simulink model "PhoenixKalman"  (R2016a)
settings: Solver=VariableStepAuto  StartTime=Seconds(firstPoint,1)  StopTime=Seconds(lastPoint,1)  RelTol=1e-3
libraries: aerolibactuator x4, aerolibanim x2, aerolib6dof2 x1, aerolibconvert2 x1
settings Model: Creator=GusBus  LastModifiedBy=GusBus
settings GRTTargetCC: GeneratePreprocessorConditionals=Use local settings

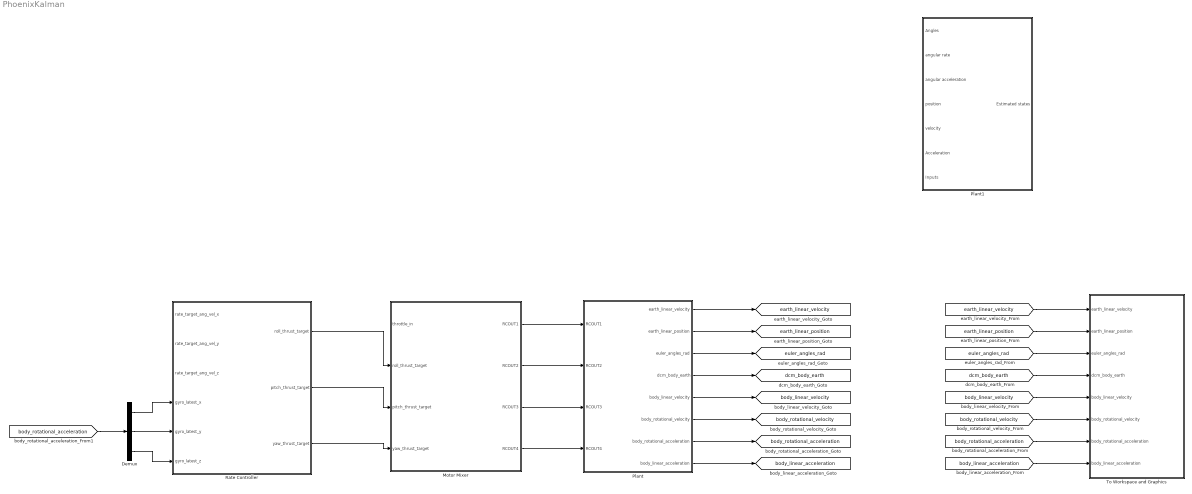
== system PhoenixKalman ==
  Demux : Demux  Outputs=3
  Motor Mixer : MATLAB Function  TreatAsAtomicUnit=on
  Plant : Subsystem
  Plant1 : Subsystem
  Rate Controller : MATLAB Function  TreatAsAtomicUnit=on
  To Workspace and Graphics : Subsystem
  tag scope: body_linear_acceleration=global, body_linear_velocity=global, body_rotational_acceleration=global, body_rotational_velocity=global, dcm_body_earth=global, earth_linear_position=global, earth_linear_velocity=global, euler_angles_rad=global
  wires:
  [body_rotational_velocity] -> To Workspace and Graphics/6(body_rotational_velocity)
  [body_linear_acceleration] -> To Workspace and Graphics/8(body_linear_acceleration)
  [body_rotational_acceleration] -> To Workspace and Graphics/7(body_rotational_acceleration)
  [body_linear_velocity] -> To Workspace and Graphics/5(body_linear_velocity)
  [dcm_body_earth] -> To Workspace and Graphics/4(dcm_body_earth)
  [euler_angles_rad] -> To Workspace and Graphics/3(euler_angles_rad)
  [earth_linear_position] -> To Workspace and Graphics/2(earth_linear_position)
  [earth_linear_velocity] -> To Workspace and Graphics/1(earth_linear_velocity)
  Plant/1(earth_linear_velocity) -> [earth_linear_velocity]
  Plant/2(earth_linear_position) -> [earth_linear_position]
  Plant/3(euler_angles_rad) -> [euler_angles_rad]
  Plant/4(dcm_body_earth) -> [dcm_body_earth]
  Plant/5(body_linear_velocity) -> [body_linear_velocity]
  Plant/6(body_rotational_velocity) -> [body_rotational_velocity]
  Plant/7(body_rotational_acceleration) -> [body_rotational_acceleration]
  Plant/8(body_linear_acceleration) -> [body_linear_acceleration]
  Motor Mixer/1(RCOUT1) -> Plant/1(RCOUT1)
  Motor Mixer/2(RCOUT2) -> Plant/2(RCOUT2)
  Motor Mixer/3(RCOUT3) -> Plant/3(RCOUT3)
  Motor Mixer/4(RCOUT4) -> Plant/4(RCOUT4)
  Rate Controller/1(roll_thrust_target) -> Motor Mixer/2(roll_thrust_target)
  Rate Controller/2(pitch_thrust_target) -> Motor Mixer/3(pitch_thrust_target)
  Rate Controller/3(yaw_thrust_target) -> Motor Mixer/4(yaw_thrust_target)
  Demux/1 -> Rate Controller/4(gyro_latest_x)
  Demux/2 -> Rate Controller/5(gyro_latest_y)
  Demux/3 -> Rate Controller/6(gyro_latest_z)
  [body_rotational_acceleration] -> Demux/1

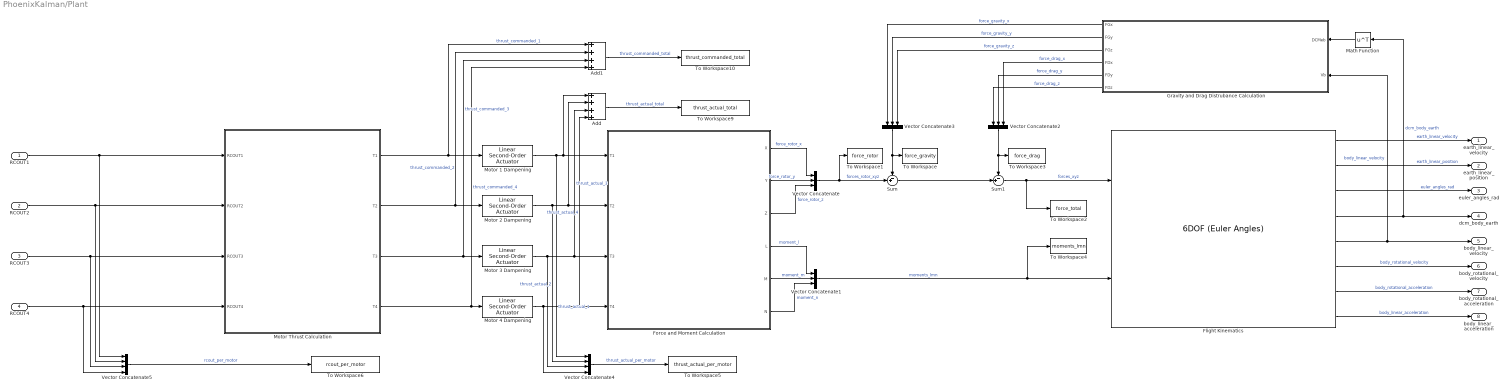
== system PhoenixKalman/Plant ==
  RCOUT1 : Inport
  RCOUT2 : Inport  Port=2
  RCOUT3 : Inport  Port=3
  RCOUT4 : Inport  Port=4
  Add : Sum  Inputs=++++
  Add1 : Sum  Inputs=++++
  Flight Kinematics : aerolib6dof2/6DOF (Euler Angles)  units=Metric (MKS)  mtype=Fixed  rep=Euler Angles  xme_0=[0 0 0]  Vm_0=[0 0 0]  eul_0=InitialAngles  pm_0=InitialRate  mass_0=2.2  mass_e=0.5  mass_f=2.0  inertia=[0.5 0 0; 0 0.5 0; 0 0 0.85]  inertia_e=eye(3)  inertia_f=2*eye(3)  k_quat=1.0  vre_flag=on
  Force and Moment Calculation : MATLAB Function  TreatAsAtomicUnit=on
  Gravity and Drag Distrubance Calculation : MATLAB Function  TreatAsAtomicUnit=on
  Math Function : Math  Operator=transpose  SaturateOnIntegerOverflow=on
  Motor 1 Dampening : aerolibactuator/Linear Second-Order Actuator  wn_fin=500  z_fin=1  fin_act_0=0  fin_act_vel=0
  Motor 2 Dampening : aerolibactuator/Linear Second-Order Actuator  wn_fin=500  z_fin=1  fin_act_0=0  fin_act_vel=0
  Motor 3 Dampening : aerolibactuator/Linear Second-Order Actuator  wn_fin=500  z_fin=1  fin_act_0=0  fin_act_vel=0
  Motor 4 Dampening : aerolibactuator/Linear Second-Order Actuator  wn_fin=500  z_fin=1  fin_act_0=0  fin_act_vel=0
  Motor Thrust Calculation : MATLAB Function  TreatAsAtomicUnit=on
  Sum : Sum  Inputs=-+|
  Sum1 : Sum  Inputs=-+|
  To Workspace : ToWorkspace  VariableName=force_gravity  SampleTime=-1
  To Workspace1 : ToWorkspace  VariableName=force_rotor  SampleTime=-1
  To Workspace10 : ToWorkspace  VariableName=thrust_commanded_total  SampleTime=-1
  To Workspace2 : ToWorkspace  VariableName=force_total  SampleTime=-1
  To Workspace3 : ToWorkspace  VariableName=force_drag  SampleTime=-1
  To Workspace4 : ToWorkspace  VariableName=moments_lmn  SampleTime=-1
  To Workspace5 : ToWorkspace  VariableName=thrust_actual_per_motor  SampleTime=-1
  To Workspace6 : ToWorkspace  VariableName=rcout_per_motor  SampleTime=-1
  To Workspace9 : ToWorkspace  VariableName=thrust_actual_total  SampleTime=-1
  Vector Concatenate{,1..3} (4 alike) : Concatenate  NumInputs=3
  Vector Concatenate4 : Concatenate  NumInputs=4
  Vector Concatenate5 : Concatenate  NumInputs=4
  earth_linear_velocity : Outport
  earth_linear_position : Outport  Port=2
  euler_angles_rad : Outport  Port=3
  dcm_body_earth : Outport  Port=4
  body_linear_velocity : Outport  Port=5
  body_rotational_velocity : Outport  Port=6
  body_rotational_acceleration : Outport  Port=7
  body_linear_acceleration : Outport  Port=8
  wires:
  Force and Moment Calculation/2(Y) -> Vector Concatenate/2  "force_rotor_y"
  Force and Moment Calculation/1(X) -> Vector Concatenate/1  "force_rotor_x"
  Force and Moment Calculation/3(Z) -> Vector Concatenate/3  "force_rotor_z"
  Force and Moment Calculation/6(N) -> Vector Concatenate1/3  "moment_n"
  Force and Moment Calculation/4(L) -> Vector Concatenate1/1  "moment_l"
  Motor Thrust Calculation/2(T2) -> Add1/2, Motor 2 Dampening/1  "thrust_commanded_2"
  Vector Concatenate1/1 -> To Workspace4/1, Flight Kinematics/2  "moments_lmn"
  Force and Moment Calculation/5(M) -> Vector Concatenate1/2  "moment_m"
  Motor 2 Dampening/1 -> Vector Concatenate4/2, Add/2, Force and Moment Calculation/2(T2)  "thrust_actual_2"
  Vector Concatenate/1 -> Sum/2, To Workspace1/1  "forces_rotor_xyz"
  Gravity and Drag Distrubance Calculation/6(FDz) -> Vector Concatenate2/1  "force_drag_z"
  Vector Concatenate3/1 -> To Workspace/1, Sum/1
  Add/1 -> To Workspace9/1  "thrust_actual_total"
  Gravity and Drag Distrubance Calculation/2(FGy) -> Vector Concatenate3/2  "force_gravity_y"
  Flight Kinematics/7 -> body_rotational_acceleration/1  "body_rotational_acceleration"
  Sum/1 -> Sum1/2
  Flight Kinematics/3 -> euler_angles_rad/1  "euler_angles_rad"
  Flight Kinematics/4 -> Math Function/1, dcm_body_earth/1  "dcm_body_earth"
  Vector Concatenate2/1 -> To Workspace3/1, Sum1/1
  Gravity and Drag Distrubance Calculation/1(FGx) -> Vector Concatenate3/1  "force_gravity_x"
  Motor Thrust Calculation/1(T1) -> Add1/1, Motor 1 Dampening/1  "thrust_commanded_1"
  Math Function/1 -> Gravity and Drag Distrubance Calculation/1(DCMeb)
  Add1/1 -> To Workspace10/1  "thrust_commanded_total"
  Motor Thrust Calculation/3(T3) -> Add1/3, Motor 3 Dampening/1  "thrust_commanded_3"
  Flight Kinematics/6 -> body_rotational_velocity/1  "body_rotational_velocity"
  Flight Kinematics/5 -> Gravity and Drag Distrubance Calculation/2(Vb), body_linear_velocity/1  "body_linear_velocity"
  Motor 1 Dampening/1 -> Vector Concatenate4/1, Add/1, Force and Moment Calculation/1(T1)  "thrust_actual_1"
  Motor 4 Dampening/1 -> Vector Concatenate4/4, Add/4, Force and Moment Calculation/4(T4)  "thrust_actual_4"
  Sum1/1 -> Flight Kinematics/1, To Workspace2/1  "forces_xyz"
  Gravity and Drag Distrubance Calculation/3(FGz) -> Vector Concatenate3/3  "force_gravity_z"
  Flight Kinematics/1 -> earth_linear_velocity/1  "earth_linear_velocity"
  Motor Thrust Calculation/4(T4) -> Add1/4, Motor 4 Dampening/1  "thrust_commanded_4"
  Gravity and Drag Distrubance Calculation/4(FDx) -> Vector Concatenate2/3  "force_drag_x"
  Gravity and Drag Distrubance Calculation/5(FDy) -> Vector Concatenate2/2  "force_drag_y"
  Flight Kinematics/8 -> body_linear_acceleration/1  "body_linear_acceleration"
  Motor 3 Dampening/1 -> Vector Concatenate4/3, Add/3, Force and Moment Calculation/3(T3)  "thrust_actual_3"
  Vector Concatenate4/1 -> To Workspace5/1  "thrust_actual_per_motor"
  Vector Concatenate5/1 -> To Workspace6/1  "rcout_per_motor"
  RCOUT1/1 -> Vector Concatenate5/1, Motor Thrust Calculation/1(RCOUT1)
  Flight Kinematics/2 -> earth_linear_position/1  "earth_linear_position"
  RCOUT2/1 -> Vector Concatenate5/2, Motor Thrust Calculation/2(RCOUT2)
  RCOUT4/1 -> Vector Concatenate5/4, Motor Thrust Calculation/4(RCOUT4)
  RCOUT3/1 -> Vector Concatenate5/3, Motor Thrust Calculation/3(RCOUT3)

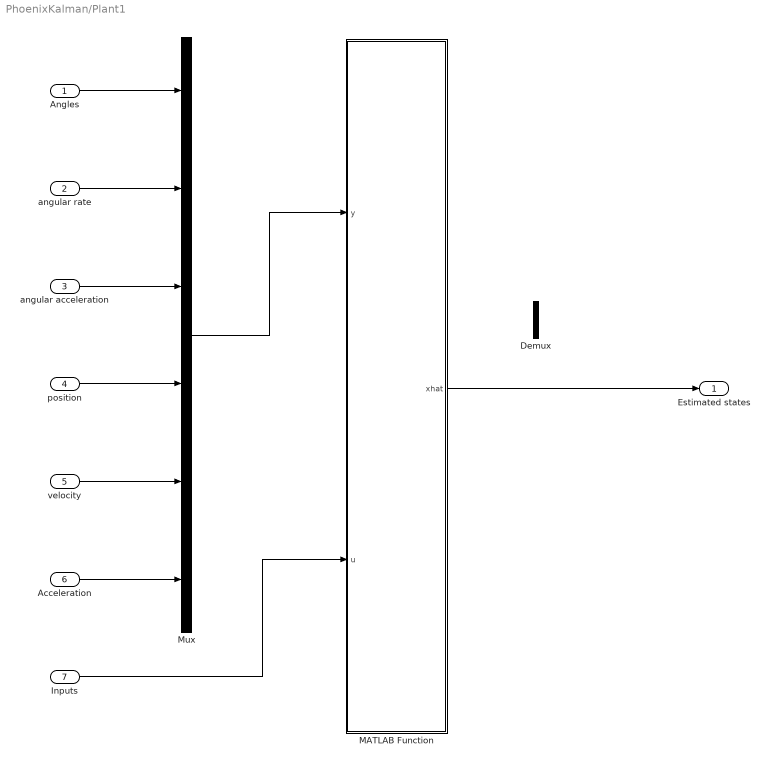
== system PhoenixKalman/Plant1 ==
  Angles : Inport
  angular rate : Inport  Port=2
  angular acceleration : Inport  Port=3
  "position " : Inport  Port=4
  velocity : Inport  Port=5
  Acceleration : Inport  Port=6
  Inputs : Inport  Port=7
  Demux : Demux  Outputs=2
  MATLAB Function : MATLAB Function  TreatAsAtomicUnit=on
  Mux : Mux  Inputs=6
  Estimated states : Outport
  wires:
  Inputs/1 -> MATLAB Function/2(u)
  Acceleration/1 -> Mux/6
  velocity/1 -> Mux/5
  "position "/1 -> Mux/4
  angular acceleration/1 -> Mux/3
  angular rate/1 -> Mux/2
  Angles/1 -> Mux/1
  Mux/1 -> MATLAB Function/1(y)
  MATLAB Function/1(xhat) -> Estimated states/1

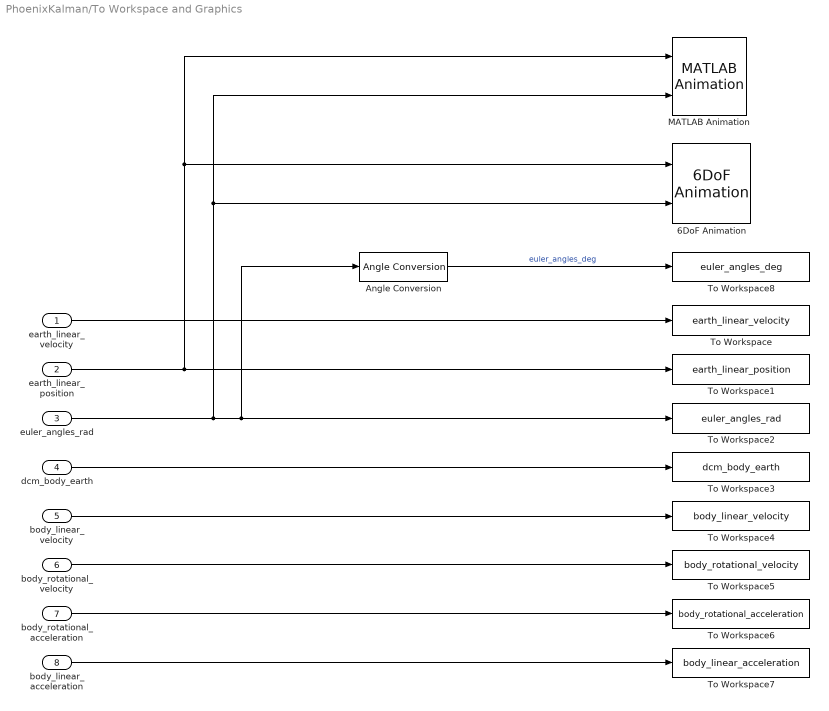
== system PhoenixKalman/To Workspace and Graphics ==
  earth_linear_velocity : Inport
  earth_linear_position : Inport  Port=2
  euler_angles_rad : Inport  Port=3
  dcm_body_earth : Inport  Port=4
  body_linear_velocity : Inport  Port=5
  body_rotational_velocity : Inport  Port=6
  body_rotational_acceleration : Inport  Port=7
  body_linear_acceleration : Inport  Port=8
  6DoF Animation : aerolibanim/6DoF Animation  u1=[0 4000 -2000 2000 -5000 -3000]  u2=0.1  u3=1.0  u4=[4000 0 -5000]  u5=Fixed position  u6=[3000 3000 3000]  u7=90  u8=off
  Angle Conversion : aerolibconvert2/Angle Conversion  IU=rad  OU=deg
  MATLAB Animation : aerolibanim/MATLAB Animation  Tag=Matlab Animation 6 DOF  Vehicles=1  Geometries='astredwedge.mat'  BoundingBoxCoordinates=[-50,50,-50,50,-50,50]  CameraOffset=[-15,-15,0]  CameraViewAngle=135  SampleTime=0.01  FigurePosition=[5,57,958,966]
  To Workspace : ToWorkspace  VariableName=earth_linear_velocity  SampleTime=-1
  To Workspace1 : ToWorkspace  VariableName=earth_linear_position  SampleTime=-1
  To Workspace2 : ToWorkspace  VariableName=euler_angles_rad  SampleTime=-1
  To Workspace3 : ToWorkspace  VariableName=dcm_body_earth  SampleTime=-1
  To Workspace4 : ToWorkspace  VariableName=body_linear_velocity  SampleTime=-1
  To Workspace5 : ToWorkspace  VariableName=body_rotational_velocity  SampleTime=-1
  To Workspace6 : ToWorkspace  VariableName=body_rotational_acceleration  SampleTime=-1
  To Workspace7 : ToWorkspace  VariableName=body_linear_acceleration  SampleTime=-1
  To Workspace8 : ToWorkspace  VariableName=euler_angles_deg  SampleTime=-1
  wires:
  body_linear_velocity/1 -> To Workspace4/1
  dcm_body_earth/1 -> To Workspace3/1
  body_rotational_velocity/1 -> To Workspace5/1
  body_linear_acceleration/1 -> To Workspace7/1
  earth_linear_position/1 -> 6DoF Animation/1, MATLAB Animation/1, To Workspace1/1
  euler_angles_rad/1 -> 6DoF Animation/2, MATLAB Animation/2, To Workspace2/1, Angle Conversion/1
  body_rotational_acceleration/1 -> To Workspace6/1
  earth_linear_velocity/1 -> To Workspace/1
  Angle Conversion/1 -> To Workspace8/1  "euler_angles_deg"

== matlab function PhoenixKalman/Plant/Motor Thrust Calculation ==
  data: RCOUT1 input; T1 output; RCOUT2 input; RCOUT3 input; RCOUT4 input; T2 output; T3 output; T4 output
function [T1, T2, T3, T4] = motorOutputs(RCOUT1, RCOUT2, RCOUT3, RCOUT4)
%   RCOUTx = PWM Value out of the Autopilot                (1000us-2000us)
%   Tx = Thrust value produced by the motor/rotor pair     (N)
%
%   1.Calculate Tmax by adding overhead onto hover throttle
%   2.Map RCOUT values between 0 and 1
%   3.Multiply unity RCOUT value by Tmax

Tmax = 2*(2.2*9.8);                                         % Overhead * (Drone3 Mass * Gravity)/number of rotors
%Tmax = 7 * 9.8 / 4;                                          % (Max Lift from website * Gravity)/number of rotors

% RCOUT1 = math_scale_values(RCOUT1, 1000, 2000, 0, 1);
% RCOUT2 = math_scale_values(RCOUT2, 1000, 2000, 0, 1);
% RCOUT3 = math_scale_values(RCOUT3, 1000, 2000, 0, 1);
% RCOUT4 = math_scale_values(RCOUT4, 1000, 2000, 0, 1);




%% Thrustprofiles

% y=a+b*x+c*x^2
a1 = 1; b1 = 2; c1 = 2;
a2 = 2; b2 = 2; c2 = 2;
a3 = 1; b3 = 2; c3 = 2;
a4 = 1; b4 = 2; c4 = 2;

Thrustprofile1 = a1+RCOUT1*b1+RCOUT1*c1;
Thrustprofile2 = a2+RCOUT2*b2+RCOUT2*c2;
Thrustprofile3 = a3+RCOUT3*b3+RCOUT3*c3;
Thrustprofile4 = a4+RCOUT4*b4+RCOUT4*c4;

T1 = Thrustprofile1*RCOUT1;
T2 = Thrustprofile2*RCOUT2;
T3 = Thrustprofile3*RCOUT3;
T4 = Thrustprofile4*RCOUT4;

%% Other ways to calculate thrust
% T1 = Tmax*RCOUT1*(0.25-0.2388+0.25);
% T2 = Tmax*RCOUT2*(0.25-0.2477+0.25);
% T3 = Tmax*RCOUT3*(0.25-0.2658+0.25);
% T4 = Tmax*RCOUT4*(0.25-0.2476+0.25);

% T1 = Tmax*RCOUT1*(0.25-0.212+0.25);
% T2 = Tmax*RCOUT2*(0.25-0.2438+0.25);
% T3 = Tmax*RCOUT3*(0.25-0.29+0.25);
% T4 = Tmax*RCOUT4*(0.25-0.2420+0.25);

% efficiencyfactor=[0.95 0.95 1 1];
% ESCfactor = [1 1 1 1];
% motorfactor = [1 1 1 1];
% 
% T1 = Tmax*RCOUT1*efficiencyfactor(1)*ESCfactor(1)*motorfactor(1);
% T2 = Tmax*RCOUT2*efficiencyfactor(2)*ESCfactor(2)*motorfactor(2);
% T3 = Tmax*RCOUT3*efficiencyfactor(3)*ESCfactor(3)*motorfactor(3);
% T4 = Tmax*RCOUT4*efficiencyfactor(4)*ESCfactor(4)*motorfactor(4);

% T1 = Tmax*RCOUT1;
% T2 = Tmax*RCOUT2;
% T3 = Tmax*RCOUT3;
% T4 = Tmax*RCOUT4;

== matlab function PhoenixKalman/Plant/Force and Moment Calculation ==
  data: T1 input; X output; T2 input; T3 input; T4 input; Y output; Z output; L output; M output; N output
function [X, Y, Z, L, M, N] = forceMomentCalc(T1, T2, T3, T4)
%T1 = Motor 1 Thrust                (N)
%T2 = Motor 2 Thrust                (N)
%T3 = Motor 3 Thrust                (N)
%T4 = Motor 4 Thrust                (N)
%X = Force in x axis                (N)
%Y = Force in y axis                (N)                
%Z = Force in z axis                (N)
%L = Rolling moment around x axis   (N.m) Forward Positive
%M = Rolling moment around y axis   (N.m) Right Positive  
%N = Rolling moment around z axis   (N.m) CW Positive

%       ccw       cw            
%X         3    1
%           \  /
%            \/
%            /\
%           /  \
%          2    4       
%       cw        ccw   Y
%%%%%%%%%%%%%%%%%%%%%%%%%
armLength = 0.41;                    %Meters
alpha = deg2rad(15);                 %Rad
chordLength = 0.040;                 %Meters
liftDragRatio = 0.1;


X = 0;
Y = 0;
Z = T1 + T2 + T3 + T4;

M = armLength * cos(alpha) * ((T2 + T4) - (T1 + T3));
L = armLength * sin(alpha) * ((T2 + T3) - (T1 + T4));
N = chordLength * ((T1 + T2) - (T3 + T4))/liftDragRatio;

== matlab function PhoenixKalman/Plant/Gravity and Drag Distrubance Calculation ==
  data: DCMeb input; FGx output; Vb input; FGy output; FGz output; FDx output; FDy output; FDz output
function [FGx, FGy, FGz, FDx, FDy, FDz] = gravityDragCalculation(DCMeb, Vb)
%   Gravity and Drag Calculations
%   Inputs
%   DCMbe = Direct Cosine Matrix, from earth to body
%   Vb = Linear Velocity, body frame
%   Outputs
%   FGa = Force of gravity in the 'a' axis, body frame
%   FDa = Force of drag in the 'a' axis, body frame

%Gravity Constants
mass = 2.2;
gravityForce_earth = [0, 0, (9.81*mass)];

%Drag Constants
airDensity = 1.1644; %wikipedia air density at 30 degrees C
dragCoefficient = 1.0; %SLADe
surfaceArea = [0.1, 0.5, 0.7]; 
Vbx = Vb(1);
Vby = Vb(2);
Vbz = Vb(3);

%Gravity Calculations
FG = gravityForce_earth * DCMeb;
FGx = FG(1);
FGy = FG(2);
FGz = FG(3);

% FGx = 0;
% FGy = 0;
% FGz = 0;

%Drag Calculations
% FDx = 0.5 * airDensity * (Vbx^2) * dragCoefficient * surfaceArea(1);
% FDy = 0.5 * airDensity * (Vby^2) * dragCoefficient * surfaceArea(2);
% FDz = 0.5 * airDensity * (Vbz^2) * dragCoefficient * surfaceArea(3);

 FDx = 0;
 FDy = 0;
 FDz = 0;


%% Trying some stupid stuff
% if Vbx > 0.000000000001
%     FDx = 0;
%     FDy = 0;
%     FDz = 0;
% else 
%     FDx = 0.5 * airDensity * (Vbx^2) * dragCoefficient * surfaceArea(1);
%     FDy = 0.5 * airDensity * (Vby^2) * dragCoefficient * surfaceArea(2);
%     FDz = 0.5 * airDensity * (Vbz^2) * dragCoefficient * surfaceArea(3);
% end

== matlab function PhoenixKalman/Rate Controller ==
  data: rate_target_ang_vel_x input; rate_target_ang_vel_y input; rate_target_ang_vel_z input; gyro_latest_x input; gyro_latest_y input; gyro_latest_z input; roll_thrust_target output; pitch_thrust_target output; yaw_thrust_target output
function [roll_thrust_target, pitch_thrust_target, yaw_thrust_target]  = rate_controller_run( rate_target_ang_vel_x, rate_target_ang_vel_y, rate_target_ang_vel_z , gyro_latest_x, gyro_latest_y, gyro_latest_z)
%RATE_CONTROLLER_RUN Summary of this function goes here
%   Detailed explanation goes here

update_throttle_rpy_mix();

roll_thrust_target = rate_target_to_motor_roll(gyro_latest_x, rate_target_ang_vel_x);

pitch_thrust_target = rate_target_to_motor_pitch(gyro_latest_y, rate_target_ang_vel_y);

yaw_thrust_target = rate_target_to_motor_yaw(gyro_latest_z, rate_target_ang_vel_z);

end

== matlab function PhoenixKalman/Motor Mixer ==
  data: throttle_in input; roll_thrust_target input; RCOUT1 output; pitch_thrust_target input; yaw_thrust_target input; RCOUT2 output; RCOUT3 output; RCOUT4 output
function [RCOUT1, RCOUT2, RCOUT3, RCOUT4 ]  = motor_mixer(throttle_in, roll_thrust_target, pitch_thrust_target, yaw_thrust_target)
%% Motor Mixer

%
%   Matlab Implementation of the ArduPilot Motor Mixer
%   Outputs Motor Commands based on required rate targets
%
%   
    global pwm_min pwm_max spin_min spin_max thrust_rpyt_out
    % Update throttle filter
    update_throttle_filter(throttle_in);

    % Update battery resistance
    % update_battery_resistance();
                                                                            %For the model, we will always assume we have maximum lift
    % Calc filtered battery voltage and lift_max
    % update_lift_max_from_batt_voltage();

    % Run spool logic
    % output_logic();
    
    % Calculate thrust
    thrust_rpyt_out = output_armed_stabilizing(roll_thrust_target, pitch_thrust_target, yaw_thrust_target);

    % Apply any thrust compensation for the frame
    % thrust_compensation();  %used for tilt rotors and tilt wings
    
    % Convert rpy_thrust values to pwm
    RCOUT1 = pwm_min + (pwm_max-pwm_min)*(spin_min + (spin_max-spin_min)*thrust_rpyt_out(1));
    RCOUT2 = pwm_min + (pwm_max-pwm_min)*(spin_min + (spin_max-spin_min)*thrust_rpyt_out(2));
    RCOUT3 = pwm_min + (pwm_max-pwm_min)*(spin_min + (spin_max-spin_min)*thrust_rpyt_out(3));
    RCOUT4 = pwm_min + (pwm_max-pwm_min)*(spin_min + (spin_max-spin_min)*thrust_rpyt_out(4));
    

end

== matlab function PhoenixKalman/Plant1/MATLAB Function ==
  data: y input; u input; xhat output
function xhat = Kalman(y,u)
%#codegen

xhat = ;
